simulink model "Solar_Inverter_Sim"  (R2021b)
settings: Solver=VariableStepAuto  StartTime=0.0  StopTime=0.8  MaxStep=1e-4  RelTol=1e-3
InitFcn:
  | run('Solar_Inverter.m');
values from neighbouring files (symbols this model uses):
  PV_Current = [3;2.99414100000000;2.98828100000000;2.98242200000000;2.97656300000000;2.97070300000000;2.96484400000000;2.95898400000000;2.95312500000000;2.94726600000000;2.94140600000000;2.93554700000000;2.92968800000000;2.92382800000000;2.91796900000000;2.91210900000000;2.90625000000000;2.90039100000000;2.89453100000000;2.88867200000000;2.88281300000000;2.87695300000000;2.87109400000000;2.86523400000000;2.8593 ...(+8480 chars)    [Solar_Inverter.m]
  PV_Voltage = [0;0.194537000000000;0.387086000000000;0.577680000000000;0.766353000000000;0.953136000000000;1.13806000000000;1.32115700000000;1.50245600000000;1.68198500000000;1.85977400000000;2.03585000000000;2.21024100000000;2.38297100000000;2.55406800000000;2.72355600000000;2.89146000000000;3.05780500000000;3.22261200000000;3.38590600000000;3.54770900000000;3.70804300000000;3.86692900000000;4.02438900000000;4 ...(+8298 chars)    [Solar_Inverter.m]
  Tc1 = 2e-5    (= 2e-05)    [Solar_Inverter.m]
  Ts1 = 2e-7    (= 2e-07)    [Solar_Inverter.m]
  Ts2 = 1e-6    (= 1e-06)    [Solar_Inverter.m]
undefined symbols (not defined in the file or in its folder): DiscIntNeverNeededParam
libraries: spsSeriesRLCBranchLib x8, spsMosfetLib x5, tiiqmathlib x4, spsCurrentMeasurementLib x3, spsPWMGeneratorDCDCLib x3, spsVoltageMeasurementLib x3, simulink x3, c28xdmclib x3, demo_controls x1, spsDiodeLib x1, spsControlledCurrentSourceLib x1, spsPowerLib x1
CloseFcn:
  | clear PV_Current PV_Voltage Ts1 Ts2 Tc1 Tc2 P_Value;
  | evalin('base', 'close(gcf)');
settings Model: SimulationMode=accelerator  Creator=The MathWorks, Inc.  LastModifiedBy=The MathWorks, Inc.
settings SolverCC: AlgebraicLoopSolver=TrustRegion
settings DataIOCC: SaveOutput=off  SaveTime=off  ReturnWorkspaceOutputs=off
settings DebuggingCC: ParameterPrecisionLossMsg=none  SFMachineParentedDataDiag=warning  ArithmeticOperatorsInVariantConditions=warning
settings SFSimCC: SimUseLocalCustomCode=off  CustomCodeUndefinedFunction=UseInterfaceOnly
settings RTWCC: RTWUseLocalCustomCode=off

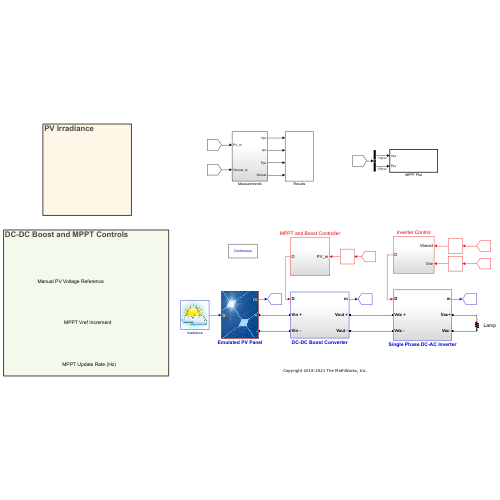
[thumbnail: Simulink's stored preview of the top-level diagram]
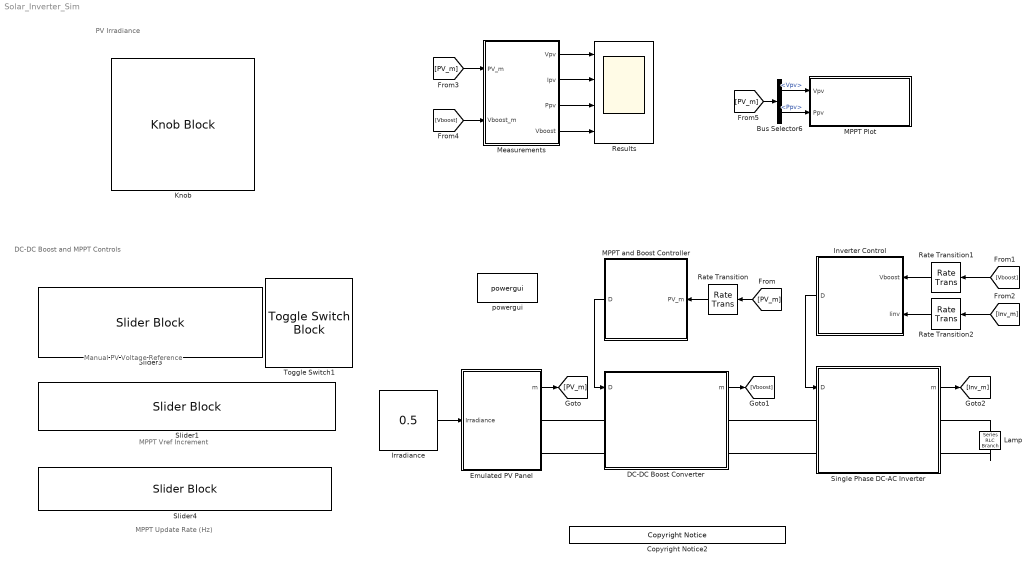
== system Solar_Inverter_Sim ==
  note: PV Irradiance
  note: DC-DC Boost and MPPT Controls
  note: MPPT Vref Increment
  note: MPPT Update Rate (Hz)
  note: Manual PV Voltage Reference
  Bus Selector6 : BusSelector  OutputSignals=Vpv,Ppv
  Copyright Notice2 : demo_controls/Copyright Notice  year=2018  prod=tic2000
      settings: SourceProductBaseCode=ME
  DC-DC Boost Converter : Subsystem
  "Emulated PV Panel " : Subsystem
      mask Display:
      | image('panel.jpg')
      | color('yellow')
      | port_label('input',1,'Ir')
      | port_label('output',1,'m')
      | port_label('Rconn',1,'+')
      | port_label('Rconn',2,'-')
  Inverter Control : Subsystem
  Irradiance : Constant  Value=0.5  OutDataTypeStr=double  SampleTime=0.05
      mask Display:
      | I = str2double(get_param('Solar_Inverter_Sim/Irradiance','Value'));
      | ud = get_param('Solar_Inverter_Sim/Irradiance','UserData');
      | if(I < 0.2)
      |     image(ud.im1);
      | elseif(I >= 0.2 && I < 0.4)
      |     image(ud.im2);
      | elseif(I >= 0.4 && I < 0.6)
      |     image(ud.im3);
      | else
      |     image(ud.im4);
      | end
  Knob : KnobBlock  ScaleMax=0.80000000000000004  TickInterval=0.10000000000000001
  Lamp : spsSeriesRLCBranchLib/Series RLC Branch  LConnTagsString=__new0  RConnTagsString=__new0  BranchType=R  Resistance=11.5  Inductance=1e-3  SetiL0=off  InitialCurrent=0  Capacitance=1e-6  Setx0=off  InitialVoltage=0  Measurements=None
  MPPT Plot : MATLAB Function  TreatAsAtomicUnit=on
  MPPT and Boost Controller : Subsystem
  Measurements : Subsystem
  Rate Transition : RateTransition  OutPortSampleTime=Tc1
  Rate Transition1 : RateTransition  OutPortSampleTime=Tc2
  Rate Transition2 : RateTransition  OutPortSampleTime=Tc2
  Results : Scope  NumInputPorts=4
  Single Phase DC-AC Inverter : Subsystem
  Slider1 : SliderBlock  ScaleMax=0.29999999999999999  TickInterval=0.050000000000000003
  Slider3 : SliderBlock  ScaleMin=1  ScaleMax=10  TickInterval=1
  Slider4 : SliderBlock  ScaleMin=25  ScaleMax=250  TickInterval=25
  Toggle Switch1 : ToggleSwitchBlock  LabelPosition=Hide
      settings: Values={{'Manual Vref', 'Enable MPPT'}, [0 1]}
  powergui : spspowerguiLib/powergui  Priority=1  SimulationMode=Continuous  SampleTime=50e-6  frequency=60  Iterations=50  frequencyindice=0  Pbase=100e6  ErrMax=1e-4  UnitsV=kV  UnitsW=MW  buscounter=0  FunctionMessages=off  echomessages=off  EnableUseOfTLC=off  CurrentSourceSwitches=off  DisableSnubberDevices=off  DisableRonSwitches=off  DisableVfSwitches=off  DisplayEquations=off  AutomaticDiscreteSolvers=off  SolverType=Tustin/Backward Euler (TBE)  Interpol=off  ExternalGateDelay=off  methode=off  Ts=100  x0status=blocks  SPID=on  SwTol=0  HookPort=off  NonlinearTolerance=1e-4  nMaxIteration=15  ContinueOnMaxIteration=off  RestoreLinks=warning  ResistiveCurrentMeasurement=off  Frange=[0:2:500]  Ylog=off  Xlog=on  ShowGrid=off  save=off  variable=ZData  structure=0  ZoomFFT=off  StartTime=0.0  cycles=1  DisplayStyle=1  fundamental=60  FreqAxis=off  MaxFrequency=1000  frequencyindicesteady=1  RmsSteady=1  display=off
  wires:
  "Emulated PV Panel "/1(m) -> [PV_m]
  [PV_m] -> Rate Transition/1
  DC-DC Boost Converter/1(m) -> [Vboost]
  Single Phase DC-AC Inverter/1(m) -> [Inv_m]
  Rate Transition/1 -> MPPT and Boost Controller/1(PV_m)
  [Vboost] -> Rate Transition1/1
  Rate Transition1/1 -> Inverter Control/1(Vboost)
  Rate Transition2/1 -> Inverter Control/2(Iinv)
  [Inv_m] -> Rate Transition2/1
  [PV_m] -> Measurements/1(PV_m)
  [Vboost] -> Measurements/2(Vboost_m)
  Measurements/1(Vpv) -> Results/1
  Measurements/2(Ipv) -> Results/2
  Measurements/3(Ppv) -> Results/3
  Measurements/4(Vboost) -> Results/4
  Bus Selector6/2 -> MPPT Plot/2(Ppv)  "<Ppv>"
  Bus Selector6/1 -> MPPT Plot/1(Vpv)  "<Vpv>"
  [PV_m] -> Bus Selector6/1
  MPPT and Boost Controller/1(D) -> DC-DC Boost Converter/1(D)
  Inverter Control/1(D) -> Single Phase DC-AC Inverter/1(D)
  Irradiance/1 -> "Emulated PV Panel "/1(Irradiance)
  connections:
  Single Phase DC-AC Inverter/LConn1 -- DC-DC Boost Converter/RConn1
  Single Phase DC-AC Inverter/LConn2 -- DC-DC Boost Converter/RConn2
  Lamp/LConn1 -- Single Phase DC-AC Inverter/RConn1
  "Emulated PV Panel "/RConn1 -- DC-DC Boost Converter/LConn1
  "Emulated PV Panel "/RConn2 -- DC-DC Boost Converter/LConn2
  Lamp/RConn1 -- Single Phase DC-AC Inverter/RConn2

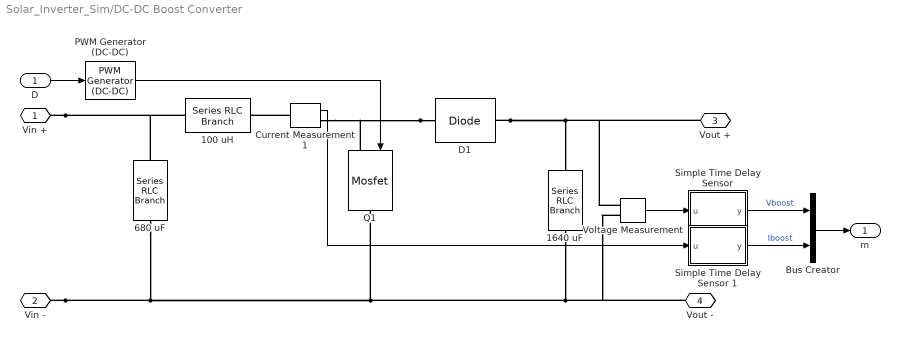
== system Solar_Inverter_Sim/DC-DC Boost Converter ==
  D : Inport
  100 uH : spsSeriesRLCBranchLib/Series RLC Branch  LConnTagsString=__new0  RConnTagsString=__new0  BranchType=L  Resistance=1  Inductance=100e-6  SetiL0=off  InitialCurrent=0  Capacitance=1e-6  Setx0=off  InitialVoltage=0  Measurements=None
  1640 uF : spsSeriesRLCBranchLib/Series RLC Branch  LConnTagsString=__new0  RConnTagsString=__new0  BranchType=C  Resistance=1  Inductance=1e-3  SetiL0=off  InitialCurrent=0  Capacitance=1640e-6  Setx0=off  InitialVoltage=30  Measurements=None
  680 uF : spsSeriesRLCBranchLib/Series RLC Branch  LConnTagsString=__new0  RConnTagsString=__new0  BranchType=C  Resistance=1  Inductance=1e-3  SetiL0=off  InitialCurrent=0  Capacitance=680e-6  Setx0=off  InitialVoltage=5  Measurements=None
  Bus Creator : BusCreator  Inputs=2
  Current Measurement1 : spsCurrentMeasurementLib/Current Measurement  PhasorSimulation=off  OutputType=Complex  PSBequivalent=0
  D1 : spsDiodeLib/Diode  Ron=0.001  Lon=0  Vf=0.8  IC=0  UseSnubber=0  Rs=500  Cs=250e-9  Measurements=off
  PWM Generator (DC-DC) : spsPWMGeneratorDCDCLib/PWM Generator (DC-DC)  Fsw=100000  Ts=Ts1
  Q1 : spsMosfetLib/Mosfet  Ron=0.1  Lon=0  Rd=0.01  Vfd=0  IC=0  Rs=1e5  Cs=inf  Measurements=off
  "Simple Time Delay Sensor " : Subsystem  mask{Ts=Ts1, Tau=0.0001}
      mask prompts: Ts "Sample Time, [s]"; Tau "Time Constant, Tau [s]"
      mask help: Simple Sensor
      mask Display: fprintf('1\n------------\n(1 + s Tau)');
  Simple Time Delay Sensor 1 : Subsystem  mask{Ts=Ts1, Tau=0.0001}
      mask prompts: Ts "Sample Time, [s]"; Tau "Time Constant, Tau [s]"
      mask help: Simple Sensor
      mask Display: fprintf('1\n------------\n(1 + s Tau)');
  Voltage Measurement : spsVoltageMeasurementLib/Voltage Measurement  PhasorSimulation=off  OutputType=Complex  PSBequivalent=0
  Vin + : PMIOPort  Side=Left
  Vin - : PMIOPort  Port=2  Side=Left
  Vout + : PMIOPort  Port=3  Side=Right
  Vout - : PMIOPort  Port=4  Side=Right
  m : Outport  VectorParamsAs1DForOutWhenUnconnected=off
  wires:
  Simple Time Delay Sensor 1/1(y) -> Bus Creator/2  "Iboost"
  "Simple Time Delay Sensor "/1(y) -> Bus Creator/1  "Vboost"
  Voltage Measurement/1 -> "Simple Time Delay Sensor "/1(u)
  Bus Creator/1 -> m/1
  Current Measurement1/1 -> Simple Time Delay Sensor 1/1(u)
  D/1 -> PWM Generator (DC-DC)/1
  PWM Generator (DC-DC)/1 -> Q1/1
  connections:
  Vin -/RConn1 -- 680 uF/RConn1 -- Vout -/RConn1 -- Voltage Measurement/LConn2 -- 1640 uF/RConn1 -- Q1/RConn1
  D1/LConn1 -- Q1/LConn1 -- Current Measurement1/RConn1
  D1/RConn1 -- 1640 uF/LConn1 -- Voltage Measurement/LConn1 -- Vout +/RConn1
  Vin +/RConn1 -- 680 uF/LConn1 -- 100 uH/LConn1
  Current Measurement1/LConn1 -- 100 uH/RConn1

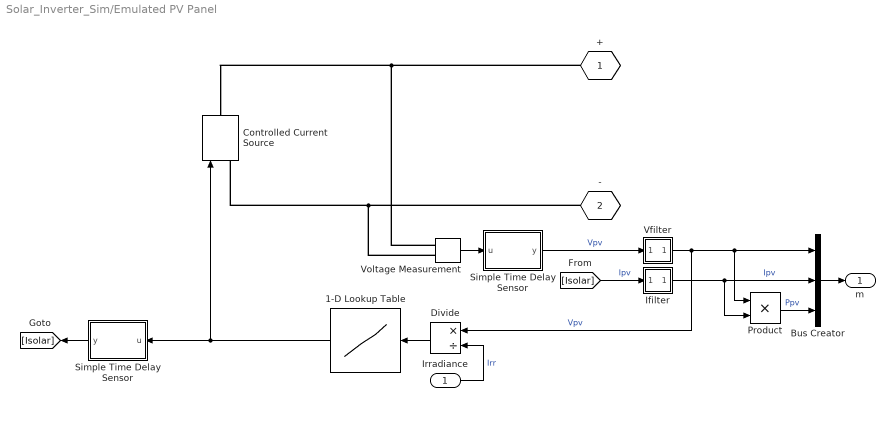
== system Solar_Inverter_Sim/Emulated PV Panel  ==
  Irradiance : Inport
  1-D Lookup Table : Lookup_n-D  NumberOfTableDimensions=1  BreakpointsForDimension1=PV_Voltage  Table=PV_Current  InternalRulePriority=Speed  RndMeth=Simplest  InputSameDT=on
  Bus Creator : BusCreator  Inputs=3
  Controlled Current Source : spsControlledCurrentSourceLib/Controlled Current Source  Initialize=on  Source_Type=DC  Amplitude=0  Phase=0  Frequency=0  Measurements=None
  Divide : Product  Inputs=*/
  Ifilter : Subsystem  mask{Tf=0.01}
      mask prompts: Tf "Filter Time Constant"
  Product : Product
  Simple Time Delay Sensor : Subsystem  mask{Ts=Ts1, Tau=0.0001}
      mask prompts: Ts "Sample Time, [s]"; Tau "Time Constant, Tau [s]"
      mask help: Simple Sensor
      mask Display: fprintf('1\n------------\n(1 + s Tau)');
  "Simple Time Delay Sensor " : Subsystem  mask{Ts=Ts1, Tau=0.0001}
      mask prompts: Ts "Sample Time, [s]"; Tau "Time Constant, Tau [s]"
      mask help: Simple Sensor
      mask Display: fprintf('1\n------------\n(1 + s Tau)');
  Vfilter : Subsystem  mask{Tf=0.01}
      mask prompts: Tf "Filter Time Constant"
  Voltage Measurement : spsVoltageMeasurementLib/Voltage Measurement  PhasorSimulation=off  OutputType=Complex  PSBequivalent=0
  + : PMIOPort  Tag=PMCPort  Side=Right
  - : PMIOPort  Tag=PMCPort  Port=2  Side=Right
  m : Outport  VectorParamsAs1DForOutWhenUnconnected=off
  wires:
  Irradiance/1 -> Divide/2  "Irr"
  Vfilter/1(y) -> Divide/1, Product/1, Bus Creator/1  "Vpv"
  Voltage Measurement/1 -> "Simple Time Delay Sensor "/1(u)
  Divide/1 -> 1-D Lookup Table/1
  Product/1 -> Bus Creator/3  "Ppv"
  Bus Creator/1 -> m/1
  Ifilter/1(y) -> Product/2, Bus Creator/2  "Ipv"
  [Isolar] -> Ifilter/1(u)  "Ipv"
  1-D Lookup Table/1 -> Controlled Current Source/1, Simple Time Delay Sensor/1(u)
  "Simple Time Delay Sensor "/1(y) -> Vfilter/1(u)  "Vpv"
  Simple Time Delay Sensor/1(y) -> [Isolar]
  connections:
  +/RConn1 -- Voltage Measurement/LConn1 -- Controlled Current Source/RConn1
  -/RConn1 -- Voltage Measurement/LConn2 -- Controlled Current Source/LConn1

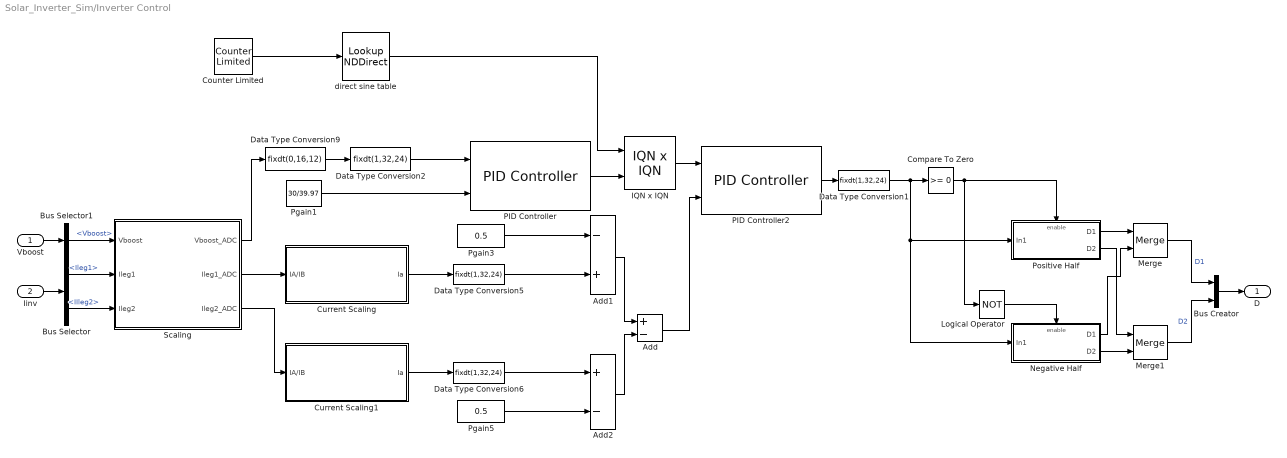
== system Solar_Inverter_Sim/Inverter Control ==
  Vboost : Inport
  Iinv : Inport  Port=2
  Add : Sum  Inputs=+-
  Add1 : Sum  Inputs=-+
  Add2 : Sum  Inputs=+-
  Bus Creator : BusCreator  Inputs=2
  Bus Selector : BusSelector  OutputSignals=Ileg1,IIleg2
  Bus Selector1 : BusSelector  OutputSignals=Vboost
  Compare To Zero : simulink/Logic and Bit Operations/Compare To Zero  relop=>=  OutDataTypeStr=boolean
  Counter Limited : simulink/Sources/Counter Limited  uplimit=400  tsamp=50e-6
  Current Scaling : Subsystem
  Current Scaling1 : Subsystem
  Data Type Conversion1 : DataTypeConversion  OutDataTypeStr=fixdt(1,32,24)
  Data Type Conversion2 : DataTypeConversion  OutDataTypeStr=fixdt(1,32,24)
  Data Type Conversion5 : DataTypeConversion  OutDataTypeStr=fixdt(1,32,24)  ConvertRealWorld=Stored Integer (SI)
  Data Type Conversion6 : DataTypeConversion  OutDataTypeStr=fixdt(1,32,24)  ConvertRealWorld=Stored Integer (SI)
  Data Type Conversion9 : DataTypeConversion  OutDataTypeStr=fixdt(0,16,12)  ConvertRealWorld=Stored Integer (SI)  RndMeth=Simplest
      settings: AttributesFormatString=DataType = %<OutDataTypeStr>
  IQN x IQN : tiiqmathlib/IQN x IQN  multiplyOption=Multiply
      settings: SourceProductBaseCode=TIC2000
  Logical Operator : Logic  Operator=NOT  AllPortsSameDT=off  OutDataTypeStr=boolean
  Merge : Merge
  Merge1 : Merge
  Negative Half : Subsystem  TreatAsAtomicUnit=on
  PID Controller : c28xdmclib/PID Controller  proportionalGain=3  integralGain=0.005  correctionGain=1  derivativeGain=0  minOutput=0  maxOutput=0.95
      settings: SourceProductBaseCode=TIC2000
  PID Controller2 : c28xdmclib/PID Controller  proportionalGain=0.25  integralGain=0.2  correctionGain=1  derivativeGain=0  minOutput=-1  maxOutput=1
      settings: SourceProductBaseCode=TIC2000
  Pgain1 : Constant  Value=30/39.97  OutDataTypeStr=fixdt(1,32,24)  SampleTime=-1
  Pgain3 : Constant  Value=0.5  OutDataTypeStr=fixdt(1,32,24)  SampleTime=50e-6
  Pgain5 : Constant  Value=0.5  OutDataTypeStr=fixdt(1,32,24)  SampleTime=50e-6
  Positive Half : Subsystem  TreatAsAtomicUnit=on
  Scaling : Subsystem
  direct sine table : LookupNDDirect  NumberOfTableDimensions=1  Table=sin( 2*pi * (0:400)/400+90/180)'  TableDataTypeStr=fixdt(1,32,24)
  D : Outport  VectorParamsAs1DForOutWhenUnconnected=off
  wires:
  PID Controller2/1 -> Data Type Conversion1/1
  Data Type Conversion1/1 -> Compare To Zero/1, Positive Half/1(In1), Negative Half/1(In1)
  Compare To Zero/1 -> Positive Half/Enable, Logical Operator/1
  Pgain3/1 -> Add1/1
  Data Type Conversion9/1 -> Data Type Conversion2/1
  IQN x IQN/1 -> PID Controller2/1
  Data Type Conversion5/1 -> Add1/2
  Positive Half/1(D1) -> Merge/1
  Add2/1 -> Add/2
  Pgain5/1 -> Add2/2
  PID Controller/1 -> IQN x IQN/2
  Pgain1/1 -> PID Controller/2
  Logical Operator/1 -> Negative Half/Enable
  Merge/1 -> Bus Creator/1  "D1"
  Merge1/1 -> Bus Creator/2  "D2"
  Current Scaling1/1(Ia) -> Data Type Conversion6/1
  Add/1 -> PID Controller2/2
  direct sine table/1 -> IQN x IQN/1
  Add1/1 -> Add/1
  Counter Limited/1 -> direct sine table/1
  Current Scaling/1(Ia) -> Data Type Conversion5/1
  Negative Half/2(D2) -> Merge1/2
  Data Type Conversion6/1 -> Add2/1
  Iinv/1 -> Bus Selector/1
  Bus Creator/1 -> D/1
  Bus Selector/2 -> Scaling/3(Ileg2)  "<IIleg2>"
  Bus Selector/1 -> Scaling/2(Ileg1)  "<Ileg1>"
  Scaling/1(Vboost_ADC) -> Data Type Conversion9/1
  Scaling/2(Ileg1_ADC) -> Current Scaling/1(IA/IB)
  Scaling/3(Ileg2_ADC) -> Current Scaling1/1(IA/IB)
  Vboost/1 -> Bus Selector1/1
  Bus Selector1/1 -> Scaling/1(Vboost)  "<Vboost>"
  Data Type Conversion2/1 -> PID Controller/1
  Positive Half/2(D2) -> Merge1/1
  Negative Half/1(D1) -> Merge/2

== system Solar_Inverter_Sim/MPPT and Boost Controller ==
  PV_m : Inport
  Bus Selector : BusSelector  OutputSignals=Vpv,Ipv
  DC-DC Boost Controller : Subsystem  TreatAsAtomicUnit=on
  MPPT : Subsystem
  Scaling and Filtering : Subsystem
  D : Outport  VectorParamsAs1DForOutWhenUnconnected=off
  wires:
  Bus Selector/1 -> Scaling and Filtering/1(Vpv)  "<Vpv>"
  Bus Selector/2 -> Scaling and Filtering/2(Ipv)  "<Ipv>"
  PV_m/1 -> Bus Selector/1
  Scaling and Filtering/2(Ipv_ADC) -> MPPT/2(Ipv)
  Scaling and Filtering/1(Vpv_ADC) -> DC-DC Boost Controller/2(Vpv), MPPT/1(Vpv)
  MPPT/1(VpvRef) -> DC-DC Boost Controller/1(VpvRef)
  DC-DC Boost Controller/1(D) -> D/1

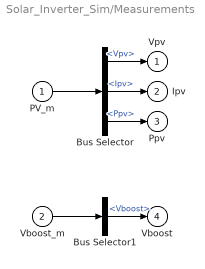
== system Solar_Inverter_Sim/Measurements ==
  PV_m : Inport
  Vboost_m : Inport  Port=2
  Bus Selector : BusSelector  OutputSignals=Vpv,Ipv,Ppv
  Bus Selector1 : BusSelector  OutputSignals=Vboost
  Vpv : Outport  VectorParamsAs1DForOutWhenUnconnected=off
  Ipv : Outport  Port=2  VectorParamsAs1DForOutWhenUnconnected=off
  Ppv : Outport  Port=3  VectorParamsAs1DForOutWhenUnconnected=off
  Vboost : Outport  Port=4  VectorParamsAs1DForOutWhenUnconnected=off
  wires:
  PV_m/1 -> Bus Selector/1
  Vboost_m/1 -> Bus Selector1/1
  Bus Selector/1 -> Vpv/1  "<Vpv>"
  Bus Selector/2 -> Ipv/1  "<Ipv>"
  Bus Selector/3 -> Ppv/1  "<Ppv>"
  Bus Selector1/1 -> Vboost/1  "<Vboost>"

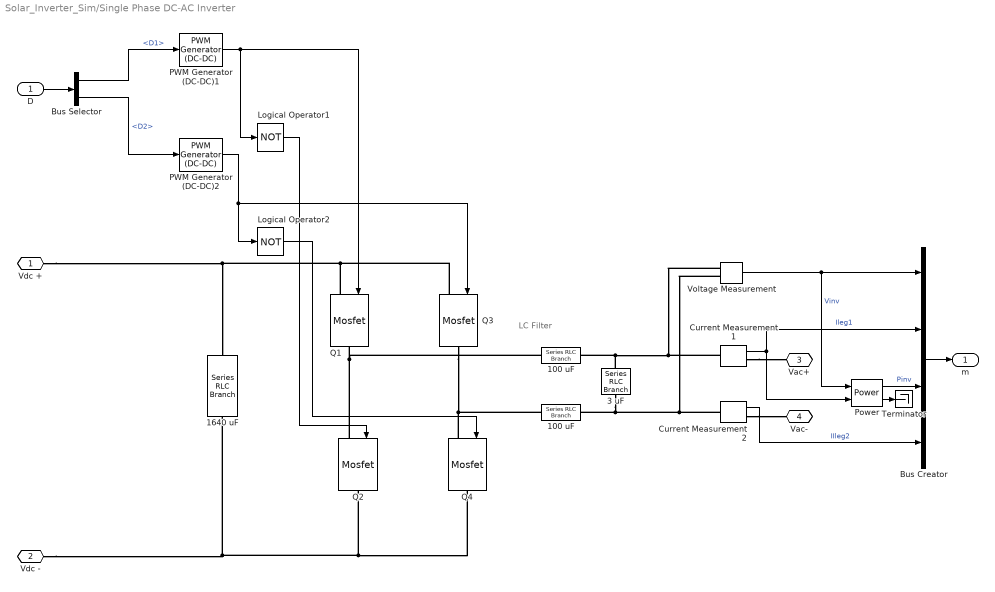
== system Solar_Inverter_Sim/Single Phase DC-AC Inverter ==
  note: LC Filter
  D : Inport
  100 uF : spsSeriesRLCBranchLib/Series RLC Branch  LConnTagsString=__new0  RConnTagsString=__new0  BranchType=L  Resistance=1  Inductance=100e-6  SetiL0=off  InitialCurrent=0  Capacitance=1e-6  Setx0=off  InitialVoltage=0  Measurements=None
  "100 uF " : spsSeriesRLCBranchLib/Series RLC Branch  LConnTagsString=__new0  RConnTagsString=__new0  BranchType=L  Resistance=1  Inductance=100e-6  SetiL0=off  InitialCurrent=0  Capacitance=1e-6  Setx0=off  InitialVoltage=0  Measurements=None
  1640 uF : spsSeriesRLCBranchLib/Series RLC Branch  LConnTagsString=__new0  RConnTagsString=__new0  BranchType=RC  Resistance=0.05  Inductance=1e-3  SetiL0=off  InitialCurrent=0  Capacitance=1640e-6  Setx0=off  InitialVoltage=0  Measurements=None
  3 uF : spsSeriesRLCBranchLib/Series RLC Branch  LConnTagsString=__new0  RConnTagsString=__new0  BranchType=C  Resistance=1  Inductance=1e-3  SetiL0=off  InitialCurrent=0  Capacitance=3e-6  Setx0=off  InitialVoltage=0  Measurements=None
  Bus Creator : BusCreator  Inputs=4
  Bus Selector : BusSelector  OutputSignals=D1,D2
  Current Measurement1 : spsCurrentMeasurementLib/Current Measurement  PhasorSimulation=off  OutputType=Complex  PSBequivalent=0
  Current Measurement2 : spsCurrentMeasurementLib/Current Measurement  PhasorSimulation=off  OutputType=Complex  PSBequivalent=0
  Logical Operator1 : Logic  Operator=NOT  AllPortsSameDT=off  OutDataTypeStr=boolean
  Logical Operator2 : Logic  Operator=NOT  AllPortsSameDT=off  OutDataTypeStr=boolean
  PWM Generator (DC-DC)1 : spsPWMGeneratorDCDCLib/PWM Generator (DC-DC)  Fsw=20000  Ts=Ts2
  PWM Generator (DC-DC)2 : spsPWMGeneratorDCDCLib/PWM Generator (DC-DC)  Fsw=20000  Ts=Ts2
  Power : spsPowerLib/Power  Freq=60  Vinit=[1, 0]  Iinit=[1, 0]  Ts=2e-3
      settings: SourceProductBaseCode=PS
  Q{1..4} (4 alike) : spsMosfetLib/Mosfet  Ron=0.1  Lon=0  Rd=0.01  Vfd=0  IC=0  Rs=1e5  Cs=inf  Measurements=off
  Terminator : Terminator
  Voltage Measurement : spsVoltageMeasurementLib/Voltage Measurement  PhasorSimulation=off  OutputType=Complex  PSBequivalent=0
  Vdc + : PMIOPort  Side=Left
  Vdc - : PMIOPort  Port=2  Side=Left
  Vac+ : PMIOPort  Port=3  Side=Right
  Vac- : PMIOPort  Port=4  Side=Right
  m : Outport  VectorParamsAs1DForOutWhenUnconnected=off
  wires:
  D/1 -> Bus Selector/1
  Voltage Measurement/1 -> Power/1, Bus Creator/1  "Vinv"
  Current Measurement1/1 -> Bus Creator/2, Power/2  "Ileg1"
  Bus Creator/1 -> m/1
  Power/1 -> Bus Creator/3  "Pinv"
  Power/2 -> Terminator/1
  Current Measurement2/1 -> Bus Creator/4  "IIleg2"
  Bus Selector/2 -> PWM Generator (DC-DC)2/1  "<D2>"
  PWM Generator (DC-DC)1/1 -> Logical Operator1/1, Q1/1
  Bus Selector/1 -> PWM Generator (DC-DC)1/1  "<D1>"
  PWM Generator (DC-DC)2/1 -> Q3/1, Logical Operator2/1
  Logical Operator1/1 -> Q2/1
  Logical Operator2/1 -> Q4/1
  connections:
  Q1/LConn1 -- Q3/LConn1 -- 1640 uF/LConn1 -- Vdc +/RConn1
  Q4/LConn1 -- Q3/RConn1 -- "100 uF "/LConn1
  Q2/LConn1 -- 100 uF/LConn1 -- Q1/RConn1
  Q2/RConn1 -- Vdc -/RConn1 -- 1640 uF/RConn1 -- Q4/RConn1
  100 uF/RConn1 -- Current Measurement1/LConn1 -- Voltage Measurement/LConn1 -- 3 uF/LConn1
  "100 uF "/RConn1 -- Current Measurement2/LConn1 -- Voltage Measurement/LConn2 -- 3 uF/RConn1
  Current Measurement1/RConn1 -- Vac+/RConn1
  Current Measurement2/RConn1 -- Vac-/RConn1

== system Solar_Inverter_Sim/DC-DC Boost Converter/Simple Time Delay Sensor  ==
  u : Inport
  1/Tau : Gain  Gain=1/Tau
  Discrete-Time Integrator : DiscreteIntegrator  SampleTime=Ts  ICPrevOutput=DiscIntNeverNeededParam  ICPrevScaledInput=DiscIntNeverNeededParam
  Sum : Sum  Inputs=|+-
  y : Outport  VectorParamsAs1DForOutWhenUnconnected=off
  wires:
  Discrete-Time Integrator/1 -> Sum/2, y/1
  u/1 -> Sum/1
  Sum/1 -> 1/Tau/1
  1/Tau/1 -> Discrete-Time Integrator/1

== system Solar_Inverter_Sim/DC-DC Boost Converter/Simple Time Delay Sensor 1 ==
  u : Inport
  1/Tau : Gain  Gain=1/Tau
  Discrete-Time Integrator : DiscreteIntegrator  SampleTime=Ts  ICPrevOutput=DiscIntNeverNeededParam  ICPrevScaledInput=DiscIntNeverNeededParam
  Sum : Sum  Inputs=|+-
  y : Outport  VectorParamsAs1DForOutWhenUnconnected=off
  wires:
  1/Tau/1 -> Discrete-Time Integrator/1
  Sum/1 -> 1/Tau/1
  u/1 -> Sum/1
  Discrete-Time Integrator/1 -> y/1, Sum/2

== system Solar_Inverter_Sim/Emulated PV Panel /Ifilter ==
  u : Inport
  1/T6 : Gain  Gain=1/Tf
  Discrete-Time Integrator : DiscreteIntegrator  SampleTime=Tc1  ICPrevOutput=DiscIntNeverNeededParam  ICPrevScaledInput=DiscIntNeverNeededParam
  Sum1 : Sum  Inputs=|+-
  y : Outport  VectorParamsAs1DForOutWhenUnconnected=off
  wires:
  Sum1/1 -> 1/T6/1
  Discrete-Time Integrator/1 -> Sum1/2, y/1
  u/1 -> Sum1/1
  1/T6/1 -> Discrete-Time Integrator/1

== system Solar_Inverter_Sim/Emulated PV Panel /Simple Time Delay Sensor ==
  u : Inport
  1/Tau : Gain  Gain=1/Tau
  Discrete-Time Integrator : DiscreteIntegrator  SampleTime=Ts  ICPrevOutput=DiscIntNeverNeededParam  ICPrevScaledInput=DiscIntNeverNeededParam
  Sum : Sum  Inputs=|+-
  y : Outport  VectorParamsAs1DForOutWhenUnconnected=off
  wires:
  1/Tau/1 -> Discrete-Time Integrator/1
  Sum/1 -> 1/Tau/1
  u/1 -> Sum/1
  Discrete-Time Integrator/1 -> y/1, Sum/2

== system Solar_Inverter_Sim/Emulated PV Panel /Simple Time Delay Sensor  ==
  u : Inport
  1/Tau : Gain  Gain=1/Tau
  Discrete-Time Integrator : DiscreteIntegrator  SampleTime=Ts  ICPrevOutput=DiscIntNeverNeededParam  ICPrevScaledInput=DiscIntNeverNeededParam
  Sum : Sum  Inputs=|+-
  y : Outport  VectorParamsAs1DForOutWhenUnconnected=off
  wires:
  Discrete-Time Integrator/1 -> Sum/2, y/1
  u/1 -> Sum/1
  Sum/1 -> 1/Tau/1
  1/Tau/1 -> Discrete-Time Integrator/1

== system Solar_Inverter_Sim/Emulated PV Panel /Vfilter ==
  u : Inport
  1/T6 : Gain  Gain=1/Tf
  Discrete-Time Integrator : DiscreteIntegrator  SampleTime=Tc1  ICPrevOutput=DiscIntNeverNeededParam  ICPrevScaledInput=DiscIntNeverNeededParam
  Sum1 : Sum  Inputs=|+-
  y : Outport  VectorParamsAs1DForOutWhenUnconnected=off
  wires:
  1/T6/1 -> Discrete-Time Integrator/1
  u/1 -> Sum1/1
  Discrete-Time Integrator/1 -> y/1, Sum1/2
  Sum1/1 -> 1/T6/1

== system Solar_Inverter_Sim/Inverter Control/Current Scaling ==
  IA/IB : Inport
  Data Type Conversion : DataTypeConversion  OutDataTypeStr=int32  ConvertRealWorld=Stored Integer (SI)
  Shift Arithmetic : ArithShift  BitShiftNumber=-12
  Ia : Outport  VectorParamsAs1DForOutWhenUnconnected=off
  wires:
  IA/IB/1 -> Data Type Conversion/1
  Shift Arithmetic/1 -> Ia/1
  Data Type Conversion/1 -> Shift Arithmetic/1

== system Solar_Inverter_Sim/Inverter Control/Current Scaling1 ==
  IA/IB : Inport
  Data Type Conversion : DataTypeConversion  OutDataTypeStr=int32  ConvertRealWorld=Stored Integer (SI)
  Shift Arithmetic : ArithShift  BitShiftNumber=-12
  Ia : Outport  VectorParamsAs1DForOutWhenUnconnected=off
  wires:
  IA/IB/1 -> Data Type Conversion/1
  Shift Arithmetic/1 -> Ia/1
  Data Type Conversion/1 -> Shift Arithmetic/1

== system Solar_Inverter_Sim/Inverter Control/Negative Half ==
  In1 : Inport
  Enable : EnablePort
  Absolute IQN : tiiqmathlib/Absolute IQN
      settings: SourceProductBaseCode=TIC2000
  Constant : Constant  Value=0  OutDataTypeStr=fixdt(1,32,24)
  D1 : Outport  VectorParamsAs1DForOutWhenUnconnected=off
  D2 : Outport  Port=2  SampleTime=50e-6  VectorParamsAs1DForOutWhenUnconnected=off
  wires:
  In1/1 -> Absolute IQN/1
  Constant/1 -> D2/1
  Absolute IQN/1 -> D1/1

== system Solar_Inverter_Sim/Inverter Control/Positive Half ==
  In1 : Inport
  Enable : EnablePort
  Constant : Constant  Value=0  OutDataTypeStr=fixdt(1,32,24)
  D1 : Outport  SampleTime=50e-6  VectorParamsAs1DForOutWhenUnconnected=off
  D2 : Outport  Port=2  VectorParamsAs1DForOutWhenUnconnected=off
  wires:
  Constant/1 -> D1/1
  In1/1 -> D2/1

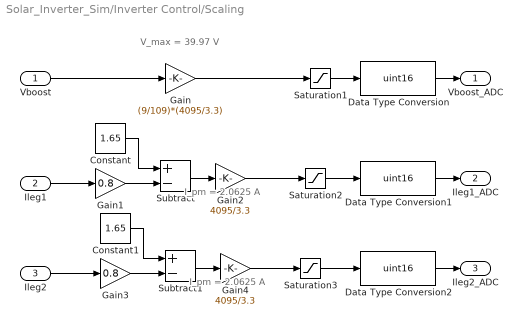
== system Solar_Inverter_Sim/Inverter Control/Scaling ==
  note: I_pm = 2.0625 A
  note: I_pm = 2.0625 A
  note: V_max = 39.97 V
  Vboost : Inport
  Ileg1 : Inport  Port=2
  Ileg2 : Inport  Port=3
  Constant : Constant  Value=1.65
  Constant1 : Constant  Value=1.65
  Data Type Conversion : DataTypeConversion  OutDataTypeStr=uint16
  Data Type Conversion1 : DataTypeConversion  OutDataTypeStr=uint16
  Data Type Conversion2 : DataTypeConversion  OutDataTypeStr=uint16
  Gain : Gain  Gain=(9/109)*(4095/3.3)
  Gain1 : Gain  Gain=0.8
  Gain2 : Gain  Gain=4095/3.3
  Gain3 : Gain  Gain=0.8
  Gain4 : Gain  Gain=4095/3.3
  Saturation1 : Saturate  UpperLimit=inf  LowerLimit=0
  Saturation2 : Saturate  UpperLimit=inf  LowerLimit=0
  Saturation3 : Saturate  UpperLimit=inf  LowerLimit=0
  Subtract : Sum  Inputs=+-
  Subtract1 : Sum  Inputs=+-
  Vboost_ADC : Outport  VectorParamsAs1DForOutWhenUnconnected=off
  Ileg1_ADC : Outport  Port=2  VectorParamsAs1DForOutWhenUnconnected=off
  Ileg2_ADC : Outport  Port=3  VectorParamsAs1DForOutWhenUnconnected=off
  wires:
  Gain2/1 -> Saturation2/1
  Constant/1 -> Subtract/1
  Gain1/1 -> Subtract/2
  Data Type Conversion1/1 -> Ileg1_ADC/1
  Subtract/1 -> Gain2/1
  Ileg1/1 -> Gain1/1
  Saturation2/1 -> Data Type Conversion1/1
  Gain3/1 -> Subtract1/2
  Ileg2/1 -> Gain3/1
  Constant1/1 -> Subtract1/1
  Subtract1/1 -> Gain4/1
  Gain4/1 -> Saturation3/1
  Saturation3/1 -> Data Type Conversion2/1
  Data Type Conversion2/1 -> Ileg2_ADC/1
  Gain/1 -> Saturation1/1
  Vboost/1 -> Gain/1
  Saturation1/1 -> Data Type Conversion/1
  Data Type Conversion/1 -> Vboost_ADC/1

== system Solar_Inverter_Sim/MPPT and Boost Controller/DC-DC Boost Controller ==
  VpvRef : Inport
  Vpv : Inport  Port=2
  DC-DC Boost Voltage Controller : c28xdmclib/PID Controller  proportionalGain=1.65  integralGain=0.0005  correctionGain=1  derivativeGain=0  minOutput=0  maxOutput=0.95
      settings: SourceProductBaseCode=TIC2000
  Data Type Conversion3 : DataTypeConversion  OutDataTypeStr=fixdt(1,32,24)
  Data Type Conversion5 : DataTypeConversion  OutDataTypeStr=fixdt(0,16,12)  ConvertRealWorld=Stored Integer (SI)  RndMeth=Simplest
      settings: AttributesFormatString=DataType = %<OutDataTypeStr>
  D : Outport  VectorParamsAs1DForOutWhenUnconnected=off
  wires:
  DC-DC Boost Voltage Controller/1 -> D/1
  Vpv/1 -> Data Type Conversion5/1
  Data Type Conversion5/1 -> Data Type Conversion3/1
  Data Type Conversion3/1 -> DC-DC Boost Voltage Controller/1
  VpvRef/1 -> DC-DC Boost Voltage Controller/2

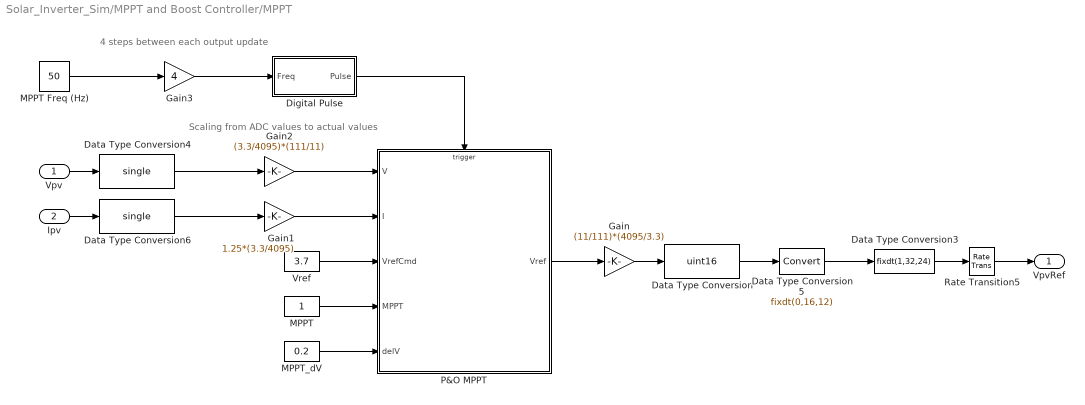
== system Solar_Inverter_Sim/MPPT and Boost Controller/MPPT ==
  note: 4 steps between each output update
  note: Scaling from ADC values to actual values
  Vpv : Inport
  Ipv : Inport  Port=2
  Data Type Conversion : DataTypeConversion  OutDataTypeStr=uint16  RndMeth=Nearest
  Data Type Conversion3 : DataTypeConversion  OutDataTypeStr=fixdt(1,32,24)
  Data Type Conversion4 : DataTypeConversion  OutDataTypeStr=single
  Data Type Conversion5 : DataTypeConversion  OutDataTypeStr=fixdt(0,16,12)  ConvertRealWorld=Stored Integer (SI)  RndMeth=Simplest
      settings: AttributesFormatString=DataType = %<OutDataTypeStr>
  Data Type Conversion6 : DataTypeConversion  OutDataTypeStr=single
  Digital Pulse : Subsystem  mask{Ts=Tc1, Duty=0.5}
      mask prompts: Ts "Sample Rate [s]"; Duty "Duty Cycle [0-1]"
  Gain : Gain  Gain=(11/111)*(4095/3.3)
  Gain1 : Gain  Gain=1.25*(3.3/4095)
  Gain2 : Gain  Gain=(3.3/4095)*(111/11)  OutDataTypeStr=single
  Gain3 : Gain  Gain=4
  MPPT : Constant  OutDataTypeStr=single  SampleTime=Tc1
  MPPT Freq (Hz) : Constant  Value=50  SampleTime=Tc1
  MPPT_dV : Constant  Value=0.2  OutDataTypeStr=single  SampleTime=Tc1
  P&O MPPT : Stateflow chart  TreatAsAtomicUnit=on
  Rate Transition5 : RateTransition  Deterministic=off  OutPortSampleTime=20e-6
  Vref : Constant  Value=3.7  OutDataTypeStr=single  SampleTime=Tc1
  VpvRef : Outport  VectorParamsAs1DForOutWhenUnconnected=off
  wires:
  P&O MPPT/1(Vref) -> Gain/1
  Vpv/1 -> Data Type Conversion4/1
  Gain1/1 -> P&O MPPT/2(I)
  Data Type Conversion/1 -> Data Type Conversion5/1
  Data Type Conversion5/1 -> Data Type Conversion3/1
  Gain/1 -> Data Type Conversion/1
  Data Type Conversion4/1 -> Gain2/1
  Ipv/1 -> Data Type Conversion6/1
  Data Type Conversion6/1 -> Gain1/1
  Gain2/1 -> P&O MPPT/1(V)
  Data Type Conversion3/1 -> Rate Transition5/1
  Rate Transition5/1 -> VpvRef/1
  Vref/1 -> P&O MPPT/3(VrefCmd)
  MPPT/1 -> P&O MPPT/4(MPPT)
  MPPT_dV/1 -> P&O MPPT/5(delV)
  MPPT Freq (Hz)/1 -> Gain3/1
  Digital Pulse/1(Pulse) -> P&O MPPT/Trigger
  Gain3/1 -> Digital Pulse/1(Freq)

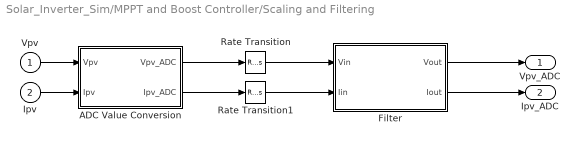
== system Solar_Inverter_Sim/MPPT and Boost Controller/Scaling and Filtering ==
  Vpv : Inport
  Ipv : Inport  Port=2
  ADC Value Conversion : Subsystem
  Filter : Subsystem
  Rate Transition : RateTransition  OutPortSampleTime=Tc1
  Rate Transition1 : RateTransition  OutPortSampleTime=Tc1
  Vpv_ADC : Outport  VectorParamsAs1DForOutWhenUnconnected=off
  Ipv_ADC : Outport  Port=2  VectorParamsAs1DForOutWhenUnconnected=off
  wires:
  Filter/2(Iout) -> Ipv_ADC/1
  Rate Transition/1 -> Filter/1(Vin)
  ADC Value Conversion/2(Ipv_ADC) -> Rate Transition1/1
  ADC Value Conversion/1(Vpv_ADC) -> Rate Transition/1
  Rate Transition1/1 -> Filter/2("Iin ")
  Vpv/1 -> ADC Value Conversion/1(Vpv)
  Ipv/1 -> ADC Value Conversion/2(Ipv)
  Filter/1(Vout) -> Vpv_ADC/1

== system Solar_Inverter_Sim/MPPT and Boost Controller/MPPT/Digital Pulse ==
  Freq : Inport
  Compare To Constant : simulink/Logic and Bit Operations/Compare To Constant  relop=>=  const=Duty  OutDataTypeStr=boolean
  Constant1 : Constant
  Discrete-Time Integrator : DiscreteIntegrator  ExternalReset=rising  SampleTime=Ts  ShowStatePort=on  ICPrevOutput=DiscIntNeverNeededParam  ICPrevScaledInput=DiscIntNeverNeededParam
  Relational Operator1 : RelationalOperator  Operator=>  OutDataTypeStr=boolean  RndMeth=Nearest
  Pulse : Outport  VectorParamsAs1DForOutWhenUnconnected=off
  wires:
  Relational Operator1/1 -> Discrete-Time Integrator/2
  Constant1/1 -> Relational Operator1/2
  Compare To Constant/1 -> Pulse/1
  Discrete-Time Integrator/State -> Relational Operator1/1
  Discrete-Time Integrator/1 -> Compare To Constant/1
  Freq/1 -> Discrete-Time Integrator/1

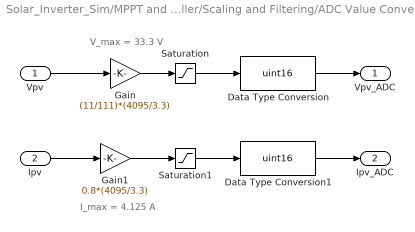
== system Solar_Inverter_Sim/MPPT and Boost Controller/Scaling and Filtering/ADC Value Conversion ==
  note: V_max = 33.3 V
  note: I_max = 4.125 A
  Vpv : Inport
  Ipv : Inport  Port=2
  Data Type Conversion : DataTypeConversion  OutDataTypeStr=uint16
  Data Type Conversion1 : DataTypeConversion  OutDataTypeStr=uint16
  Gain : Gain  Gain=(11/111)*(4095/3.3)
  Gain1 : Gain  Gain=0.8*(4095/3.3)
  Saturation : Saturate  UpperLimit=inf  LowerLimit=0
  Saturation1 : Saturate  UpperLimit=inf  LowerLimit=0
  Vpv_ADC : Outport  VectorParamsAs1DForOutWhenUnconnected=off
  Ipv_ADC : Outport  Port=2  VectorParamsAs1DForOutWhenUnconnected=off
  wires:
  Vpv/1 -> Gain/1
  Ipv/1 -> Gain1/1
  Gain/1 -> Saturation/1
  Gain1/1 -> Saturation1/1
  Data Type Conversion/1 -> Vpv_ADC/1
  Data Type Conversion1/1 -> Ipv_ADC/1
  Saturation/1 -> Data Type Conversion/1
  Saturation1/1 -> Data Type Conversion1/1

== system Solar_Inverter_Sim/MPPT and Boost Controller/Scaling and Filtering/Filter ==
  Vin : Inport
  "Iin " : Inport  Port=2
  EMA : Subsystem
  EMA1 : Subsystem
  Vout : Outport  VectorParamsAs1DForOutWhenUnconnected=off
  Iout : Outport  Port=2  VectorParamsAs1DForOutWhenUnconnected=off
  wires:
  Vin/1 -> EMA/1(In1)
  EMA/1(Out1) -> Vout/1
  "Iin "/1 -> EMA1/1(In1)
  EMA1/1(Out1) -> Iout/1

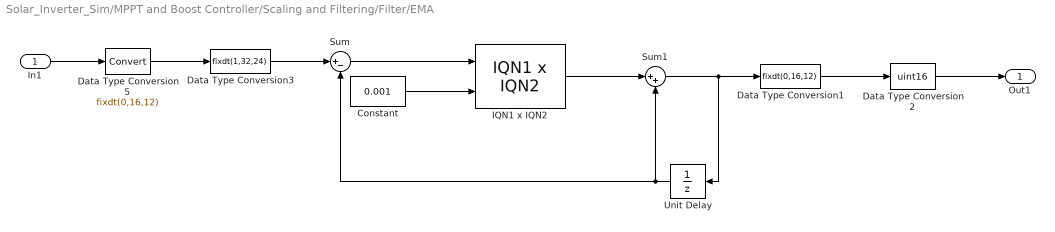
== system Solar_Inverter_Sim/MPPT and Boost Controller/Scaling and Filtering/Filter/EMA ==
  In1 : Inport  OutDataTypeStr=uint16
  Constant : Constant  Value=0.001  OutDataTypeStr=fixdt(1,32,30)
  Data Type Conversion1 : DataTypeConversion  OutDataTypeStr=fixdt(0,16,12)
  Data Type Conversion2 : DataTypeConversion  OutDataTypeStr=uint16  ConvertRealWorld=Stored Integer (SI)  RndMeth=Simplest
      settings: AttributesFormatString=DataType = %<OutDataTypeStr>
  Data Type Conversion3 : DataTypeConversion  OutDataTypeStr=fixdt(1,32,24)
  Data Type Conversion5 : DataTypeConversion  OutDataTypeStr=fixdt(0,16,12)  ConvertRealWorld=Stored Integer (SI)  RndMeth=Simplest
      settings: AttributesFormatString=DataType = %<OutDataTypeStr>
  IQN1 x IQN2 : tiiqmathlib/IQN1 x IQN2  Q=24
      settings: SourceProductBaseCode=TIC2000
  Sum : Sum  Inputs=|+-  OutDataTypeStr=fixdt(1,32,24)
  Sum1 : Sum  Inputs=|++
  Unit Delay : UnitDelay  SampleTime=-1  HasFrameUpgradeWarning=on
  Out1 : Outport  OutDataTypeStr=uint16  VectorParamsAs1DForOutWhenUnconnected=off
  wires:
  Sum/1 -> IQN1 x IQN2/1
  IQN1 x IQN2/1 -> Sum1/1
  Sum1/1 -> Unit Delay/1, Data Type Conversion1/1
  Unit Delay/1 -> Sum/2, Sum1/2
  Constant/1 -> IQN1 x IQN2/2
  Data Type Conversion5/1 -> Data Type Conversion3/1
  In1/1 -> Data Type Conversion5/1
  Data Type Conversion3/1 -> Sum/1
  Data Type Conversion1/1 -> Data Type Conversion2/1
  Data Type Conversion2/1 -> Out1/1

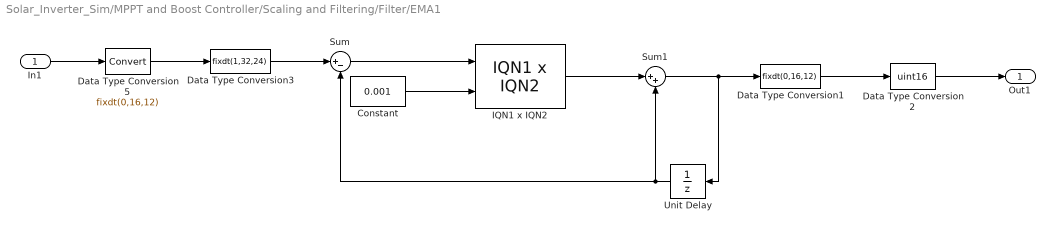
== system Solar_Inverter_Sim/MPPT and Boost Controller/Scaling and Filtering/Filter/EMA1 ==
  In1 : Inport  OutDataTypeStr=uint16
  Constant : Constant  Value=0.001  OutDataTypeStr=fixdt(1,32,30)
  Data Type Conversion1 : DataTypeConversion  OutDataTypeStr=fixdt(0,16,12)
  Data Type Conversion2 : DataTypeConversion  OutDataTypeStr=uint16  ConvertRealWorld=Stored Integer (SI)  RndMeth=Simplest
      settings: AttributesFormatString=DataType = %<OutDataTypeStr>
  Data Type Conversion3 : DataTypeConversion  OutDataTypeStr=fixdt(1,32,24)
  Data Type Conversion5 : DataTypeConversion  OutDataTypeStr=fixdt(0,16,12)  ConvertRealWorld=Stored Integer (SI)  RndMeth=Simplest
      settings: AttributesFormatString=DataType = %<OutDataTypeStr>
  IQN1 x IQN2 : tiiqmathlib/IQN1 x IQN2  Q=24
      settings: SourceProductBaseCode=TIC2000
  Sum : Sum  Inputs=|+-  OutDataTypeStr=fixdt(1,32,24)
  Sum1 : Sum  Inputs=|++
  Unit Delay : UnitDelay  SampleTime=-1  HasFrameUpgradeWarning=on
  Out1 : Outport  OutDataTypeStr=uint16  VectorParamsAs1DForOutWhenUnconnected=off
  wires:
  Data Type Conversion2/1 -> Out1/1
  Data Type Conversion1/1 -> Data Type Conversion2/1
  Data Type Conversion3/1 -> Sum/1
  In1/1 -> Data Type Conversion5/1
  Data Type Conversion5/1 -> Data Type Conversion3/1
  Constant/1 -> IQN1 x IQN2/2
  Unit Delay/1 -> Sum1/2, Sum/2
  Sum1/1 -> Data Type Conversion1/1, Unit Delay/1
  IQN1 x IQN2/1 -> Sum1/1
  Sum/1 -> IQN1 x IQN2/1

== stateflow chart Solar_Inverter_Sim/MPPT and Boost Controller/MPPT/P&O MPPT ==
  settings: executeAtInitialization=1
  state DisableMPPT
    during:
    Vref = VrefCmd;
    Vref_prev = VrefCmd;
  state EnableMPPT
    state WAIT
    state INIT
      du:
      C = C+1;
    state Compute_Power
      entry:
      P = V*I;
    state Calculate_Difference
      entry:
      deltaP = P - Pprev;
      deltaV = V - Vprev;
    state Decrement_Vref
      entry:
      Vref = Vref_prev - delV;
    state Increment_Vref
      entry:
      Vref = Vref_prev + delV;
    state Save_PreviousValues
      entry:
      Pprev = P; Vprev = V;
    state Clamp_VrefMax
      entry:
      Vref = VrefMax;
    state Clamp_VrefMin
      entry:
      Vref = VrefMin;
    (default) -> WAIT
    WAIT -> INIT : {C = 0;}
    INIT -> Compute_Power : [C == 1]{Vref_prev = 0.8*V;}
    (junction 96) -> Compute_Power
    (junction 106) -> (junction 96) : {Vref_prev = Vref;}
    Compute_Power -> Calculate_Difference
    Calculate_Difference -> (junction 103) [order 1] : [deltaP < 0]
    Calculate_Difference -> (junction 104) [order 2] : [deltaP >= 0]
    (junction 103) -> Increment_Vref [order 2] : [deltaV < 0]
    (junction 104) -> Decrement_Vref [order 1] : [deltaV <= 0]
    (junction 103) -> Decrement_Vref [order 1] : [deltaV >= 0]
    (junction 104) -> Increment_Vref [order 2] : [deltaV > 0]
    Decrement_Vref -> Save_PreviousValues
    Increment_Vref -> Save_PreviousValues
    Save_PreviousValues -> (junction 106) [order 3]
    (junction 73) -> (junction 106)
    Save_PreviousValues -> Clamp_VrefMax [order 1] : [Vref >= VrefMax]
    Save_PreviousValues -> Clamp_VrefMin [order 2] : [Vref <= VrefMin]
    Clamp_VrefMax -> (junction 88)
    Clamp_VrefMin -> (junction 98)
    (junction 88) -> (junction 98)
    (junction 98) -> (junction 73)
  (default) -> DisableMPPT
  (junction 89) -> DisableMPPT
  EnableMPPT -> (junction 89) : [MPPT ~= 1]
  DisableMPPT -> EnableMPPT : [MPPT == 1 && V>=4]
  data: P local single =single(0); deltaP local single =single(0); Pprev local single =single(0); Vprev local single =single(0); deltaV local single =single(0); V input; I input; Vref output single; Vref_prev local; C local; VrefCmd input; MPPT input; delV input single; VrefMax constant single =single(28); VrefMin constant single =single(1)
  events: event input RISING_EDGE_EVENT

== matlab function Solar_Inverter_Sim/MPPT Plot ==
  data: Vpv input; Ppv input; PV_Voltage parameter; PV_Current parameter
function plotPVPower(Vpv,Ppv,PV_Voltage,PV_Current)

    persistent irrPlot powerPlot
%     coder.extrinsic('legend');   

    Irr = [0.2,0.3,0.4,0.5,0.6,0.7,0.8];

    if isempty(irrPlot)
                        
        figure(1);
        for i = 1: length(Irr)
            irrPlot = plot(PV_Voltage*Irr(i),Irr(i)*(PV_Voltage.*PV_Current));hold on;
        end
        grid on;
        
        xlabel('PV Voltage [V]');
        ylabel('PV Power [W]');
        title('PV Power Output');
        
        powerPlot = plot(Vpv,Ppv,'ro'); 
        %legend('100 W/m^2','200 W/m^2','300 W/m^2','400 W/m^2','500 W/m^2','600 W/m^2','700 W/m^2','800 W/m^2','PV Power');
        
        hold off;

    else 
        set(powerPlot,'XData',Vpv,'YData',Ppv);
    end
    
end
